simulink model "model3_ReferenceInput"  (R2020a)
settings: Solver=FixedStepAuto  StartTime=0.0  StopTime=T  FixedStep=Ts  RelTol=1e-3
undefined symbols (not defined in the file): K, L, M, N, omgn, R, stepT, Ts, x0
settings Model: Creator=XiaoCY  LastModifiedBy=XiaoCY
settings DataIOCC: ReturnWorkspaceOutputs=off

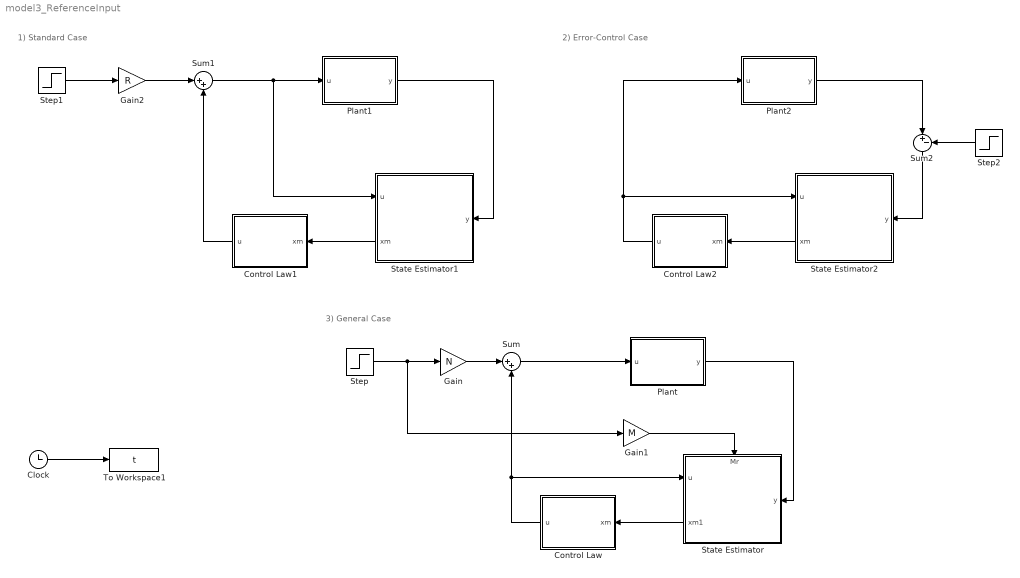
== system model3_ReferenceInput ==
  note: 3) General Case
  note: 1) Standard Case
  note: 2) Error-Control Case
  Clock : Clock
  Control Law : Subsystem
  Control Law1 : Subsystem
  Control Law2 : Subsystem
  Gain : Gain  Gain=N
  Gain1 : Gain  Gain=M
  Gain2 : Gain  Gain=R
  Plant : Subsystem
  Plant1 : Subsystem
  Plant2 : Subsystem
  State Estimator : Subsystem
      settings: PortSchema="{\"entries\":[{\"content\":{\"sides\":[{\"content\":{\"connectorIds\":[\"In1\"]},\"type\":\"ConnectorPlacement.EquallySpacedRectSide\",\"uuid\":\"995efd48-3db5-4a6e-85f6-a349d6a63930\"},{\"content\":{\"connectorIds\":[\"In3\",\"Out1\"],\"side\":\"RIGHT\"},\"type\":\"ConnectorPlacement.EquallySpacedRectSide\",\"uuid\":\"626e22d4-5752-4239-b2ce-472c77ace920\"},{\"content\":{\"connectorIds\":[\"In2\"],\"side\":\"TOP\"},\"type\":\"ConnectorPlacement.EquallySpacedRectSide\",\"uuid\":\"cb599412-420c-4014-940e-49f432b7cbea\"}]},\"type\":\"ConnectorPlacement.EquallySpacedConnector\",\"uuid\":\"e0cccee1-86a0-41f4-a3e5-9044b1b28e69\"}],\"packageUris\":[\"http://schema.mathworks.com/mf0/Connector/19700101\"],\"version\":\"1.0\"}"
  State Estimator1 : Subsystem
      settings: PortSchema="{\"entries\":[{\"content\":{\"sides\":[{\"content\":{\"connectorIds\":[\"In1\"]},\"type\":\"ConnectorPlacement.EquallySpacedRectSide\",\"uuid\":\"995efd48-3db5-4a6e-85f6-a349d6a63930\"},{\"content\":{\"connectorIds\":[\"In2\",\"Out1\"],\"side\":\"RIGHT\"},\"type\":\"ConnectorPlacement.EquallySpacedRectSide\",\"uuid\":\"626e22d4-5752-4239-b2ce-472c77ace920\"},{\"content\":{\"connectorIds\":[],\"side\":\"TOP\"},\"type\":\"ConnectorPlacement.EquallySpacedRectSide\",\"uuid\":\"cb599412-420c-4014-940e-49f432b7cbea\"}]},\"type\":\"ConnectorPlacement.EquallySpacedConnector\",\"uuid\":\"e0cccee1-86a0-41f4-a3e5-9044b1b28e69\"}],\"packageUris\":[\"http://schema.mathworks.com/mf0/Connector/19700101\"],\"version\":\"1.0\"}"
  State Estimator2 : Subsystem
      settings: PortSchema="{\"entries\":[{\"content\":{\"sides\":[{\"content\":{\"connectorIds\":[\"In1\"]},\"type\":\"ConnectorPlacement.EquallySpacedRectSide\",\"uuid\":\"995efd48-3db5-4a6e-85f6-a349d6a63930\"},{\"content\":{\"connectorIds\":[\"In2\",\"Out1\"],\"side\":\"RIGHT\"},\"type\":\"ConnectorPlacement.EquallySpacedRectSide\",\"uuid\":\"626e22d4-5752-4239-b2ce-472c77ace920\"},{\"content\":{\"connectorIds\":[],\"side\":\"TOP\"},\"type\":\"ConnectorPlacement.EquallySpacedRectSide\",\"uuid\":\"cb599412-420c-4014-940e-49f432b7cbea\"}]},\"type\":\"ConnectorPlacement.EquallySpacedConnector\",\"uuid\":\"e0cccee1-86a0-41f4-a3e5-9044b1b28e69\"}],\"packageUris\":[\"http://schema.mathworks.com/mf0/Connector/19700101\"],\"version\":\"1.0\"}"
  Step : Step  Time=stepT  SampleTime=0
  Step1 : Step  Time=stepT  SampleTime=0
  Step2 : Step  Time=stepT  SampleTime=0
  Sum : Sum  Inputs=|++
  Sum1 : Sum  Inputs=|++
  Sum2 : Sum  Inputs=|+-
  To Workspace1 : ToWorkspace  VariableName=t  SampleTime=Ts
  wires:
  Clock/1 -> To Workspace1/1
  Plant/1(y) -> State Estimator/1(y)
  State Estimator/1(xm1) -> Control Law/1(xm)
  Control Law/1(u) -> State Estimator/3(u), Sum/2
  Step/1 -> Gain1/1, Gain/1
  Sum/1 -> Plant/1(u)
  Gain/1 -> Sum/1
  Gain1/1 -> State Estimator/2(Mr)
  Gain2/1 -> Sum1/1
  Sum1/1 -> State Estimator1/2(u), Plant1/1(u)
  Step1/1 -> Gain2/1
  Control Law1/1(u) -> Sum1/2
  State Estimator1/1(xm) -> Control Law1/1(xm)
  Plant1/1(y) -> State Estimator1/1(y)
  State Estimator2/1(xm) -> Control Law2/1(xm)
  Control Law2/1(u) -> Plant2/1(u), State Estimator2/2(u)
  Plant2/1(y) -> Sum2/1
  Sum2/1 -> State Estimator2/1(y)
  Step2/1 -> Sum2/2

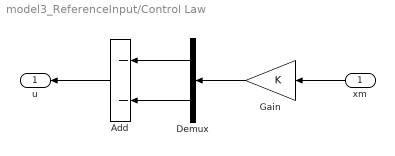
== system model3_ReferenceInput/Control Law ==
  xm : Inport
  Add : Sum  Inputs=--
  Demux : Demux  Outputs=2
  Gain : Gain  Gain=K
  u : Outport
  wires:
  xm/1 -> Gain/1
  Demux/2 -> Add/2
  Add/1 -> u/1
  Gain/1 -> Demux/1
  Demux/1 -> Add/1

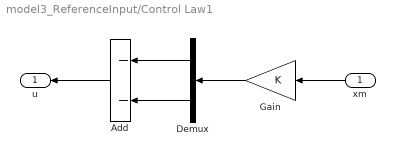
== system model3_ReferenceInput/Control Law1 ==
  xm : Inport
  Add : Sum  Inputs=--
  Demux : Demux  Outputs=2
  Gain : Gain  Gain=K
  u : Outport
  wires:
  Demux/1 -> Add/1
  Gain/1 -> Demux/1
  Add/1 -> u/1
  Demux/2 -> Add/2
  xm/1 -> Gain/1

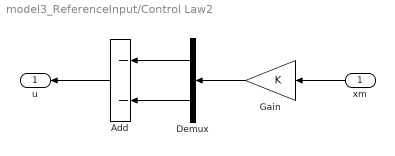
== system model3_ReferenceInput/Control Law2 ==
  xm : Inport
  Add : Sum  Inputs=--
  Demux : Demux  Outputs=2
  Gain : Gain  Gain=K
  u : Outport
  wires:
  xm/1 -> Gain/1
  Demux/2 -> Add/2
  Add/1 -> u/1
  Gain/1 -> Demux/1
  Demux/1 -> Add/1

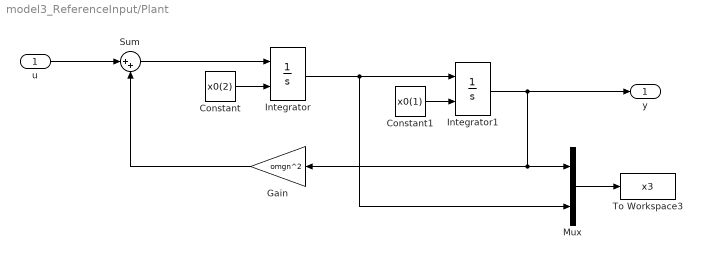
== system model3_ReferenceInput/Plant ==
  u : Inport
  Constant : Constant  Value=x0(2)
  Constant1 : Constant  Value=x0(1)
  Gain : Gain  Gain=omgn^2
  Integrator : Integrator  InitialConditionSource=external
  Integrator1 : Integrator  InitialConditionSource=external
  Mux : Mux  Inputs=2
  Sum : Sum  Inputs=|++
  To Workspace3 : ToWorkspace  VariableName=x3  SampleTime=Ts
  y : Outport
  wires:
  Integrator/1 -> Mux/2, Integrator1/1
  Constant1/1 -> Integrator1/2
  u/1 -> Sum/1
  Constant/1 -> Integrator/2
  Sum/1 -> Integrator/1
  Gain/1 -> Sum/2
  Mux/1 -> To Workspace3/1
  Integrator1/1 -> Gain/1, Mux/1, y/1

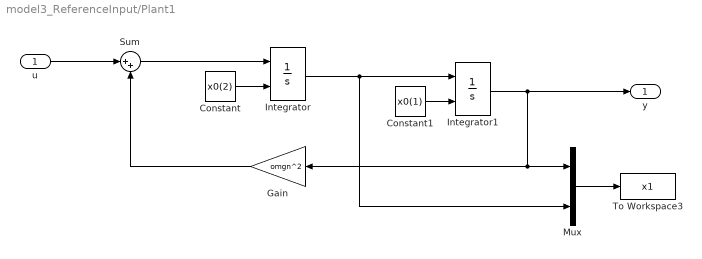
== system model3_ReferenceInput/Plant1 ==
  u : Inport
  Constant : Constant  Value=x0(2)
  Constant1 : Constant  Value=x0(1)
  Gain : Gain  Gain=omgn^2
  Integrator : Integrator  InitialConditionSource=external
  Integrator1 : Integrator  InitialConditionSource=external
  Mux : Mux  Inputs=2
  Sum : Sum  Inputs=|++
  To Workspace3 : ToWorkspace  VariableName=x1  SampleTime=Ts
  y : Outport
  wires:
  Integrator1/1 -> y/1, Mux/1, Gain/1
  Mux/1 -> To Workspace3/1
  Gain/1 -> Sum/2
  Sum/1 -> Integrator/1
  Constant/1 -> Integrator/2
  u/1 -> Sum/1
  Constant1/1 -> Integrator1/2
  Integrator/1 -> Integrator1/1, Mux/2

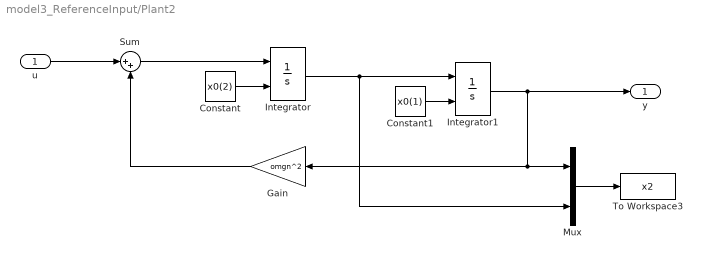
== system model3_ReferenceInput/Plant2 ==
  u : Inport
  Constant : Constant  Value=x0(2)
  Constant1 : Constant  Value=x0(1)
  Gain : Gain  Gain=omgn^2
  Integrator : Integrator  InitialConditionSource=external
  Integrator1 : Integrator  InitialConditionSource=external
  Mux : Mux  Inputs=2
  Sum : Sum  Inputs=|++
  To Workspace3 : ToWorkspace  VariableName=x2  SampleTime=Ts
  y : Outport
  wires:
  Integrator/1 -> Mux/2, Integrator1/1
  Constant1/1 -> Integrator1/2
  u/1 -> Sum/1
  Constant/1 -> Integrator/2
  Sum/1 -> Integrator/1
  Gain/1 -> Sum/2
  Mux/1 -> To Workspace3/1
  Integrator1/1 -> Gain/1, Mux/1, y/1

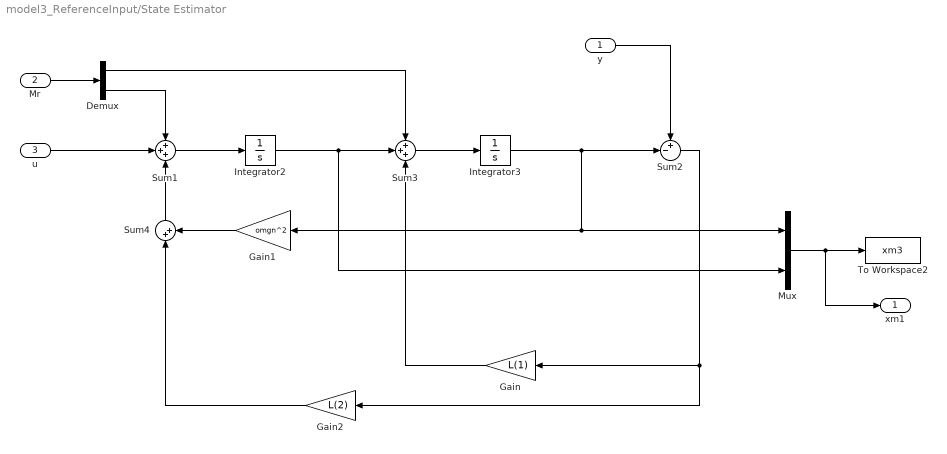
== system model3_ReferenceInput/State Estimator ==
  y : Inport
  Mr : Inport  Port=2
  u : Inport  Port=3
  Demux : Demux  Outputs=2
  Gain : Gain  Gain=L(1)
  Gain1 : Gain  Gain=omgn^2
  Gain2 : Gain  Gain=L(2)
  Integrator2 : Integrator
  Integrator3 : Integrator
  Mux : Mux  Inputs=2
  Sum1 : Sum  Inputs=+++
  Sum2 : Sum  Inputs=+-|
  Sum3 : Sum  Inputs=+++
  Sum4 : Sum  Inputs=|++
  To Workspace2 : ToWorkspace  VariableName=xm3  SampleTime=Ts
  xm1 : Outport
  wires:
  y/1 -> Sum2/1
  Integrator3/1 -> Sum2/2, Mux/1, Gain1/1
  Sum1/1 -> Integrator2/1
  u/1 -> Sum1/2
  Integrator2/1 -> Sum3/2, Mux/2
  Mux/1 -> xm1/1, To Workspace2/1
  Sum2/1 -> Gain2/1, Gain/1
  Sum3/1 -> Integrator3/1
  Gain1/1 -> Sum4/2
  Sum4/1 -> Sum1/3
  Gain/1 -> Sum3/3
  Gain2/1 -> Sum4/1
  Mr/1 -> Demux/1
  Demux/1 -> Sum3/1
  Demux/2 -> Sum1/1

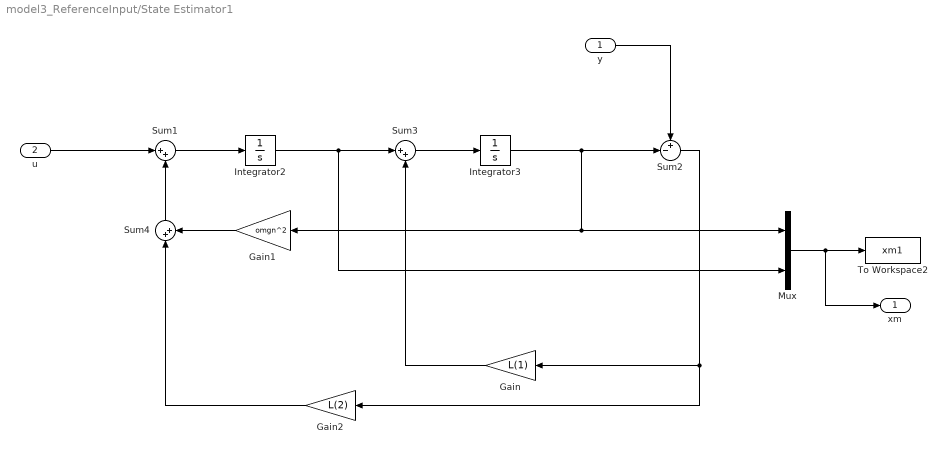
== system model3_ReferenceInput/State Estimator1 ==
  y : Inport
  u : Inport  Port=2
  Gain : Gain  Gain=L(1)
  Gain1 : Gain  Gain=omgn^2
  Gain2 : Gain  Gain=L(2)
  Integrator2 : Integrator
  Integrator3 : Integrator
  Mux : Mux  Inputs=2
  Sum1 : Sum  Inputs=|++
  Sum2 : Sum  Inputs=+-|
  Sum3 : Sum  Inputs=|++
  Sum4 : Sum  Inputs=|++
  To Workspace2 : ToWorkspace  VariableName=xm1  SampleTime=Ts
  xm : Outport
  wires:
  Gain2/1 -> Sum4/1
  Gain/1 -> Sum3/2
  Sum4/1 -> Sum1/2
  Gain1/1 -> Sum4/2
  Sum3/1 -> Integrator3/1
  Sum2/1 -> Gain/1, Gain2/1
  Mux/1 -> To Workspace2/1, xm/1
  Integrator2/1 -> Sum3/1, Mux/2
  u/1 -> Sum1/1
  Sum1/1 -> Integrator2/1
  Integrator3/1 -> Gain1/1, Mux/1, Sum2/2
  y/1 -> Sum2/1

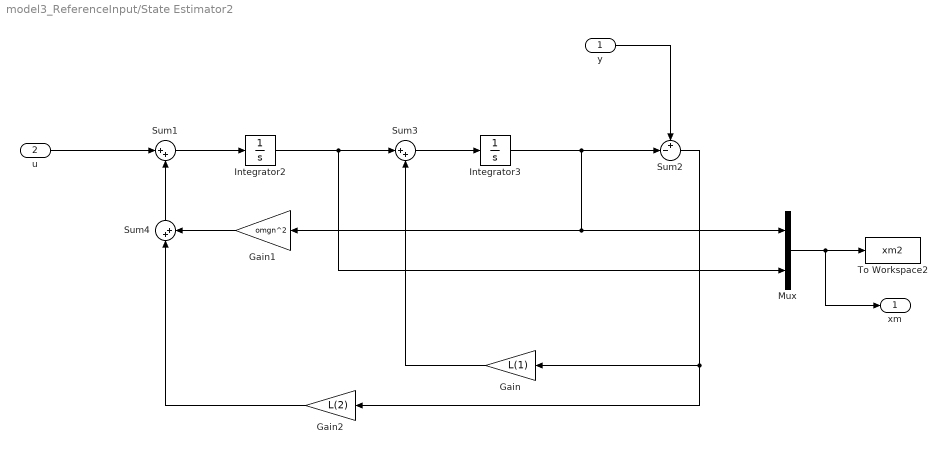
== system model3_ReferenceInput/State Estimator2 ==
  y : Inport
  u : Inport  Port=2
  Gain : Gain  Gain=L(1)
  Gain1 : Gain  Gain=omgn^2
  Gain2 : Gain  Gain=L(2)
  Integrator2 : Integrator
  Integrator3 : Integrator
  Mux : Mux  Inputs=2
  Sum1 : Sum  Inputs=|++
  Sum2 : Sum  Inputs=+-|
  Sum3 : Sum  Inputs=|++
  Sum4 : Sum  Inputs=|++
  To Workspace2 : ToWorkspace  VariableName=xm2  SampleTime=Ts
  xm : Outport
  wires:
  y/1 -> Sum2/1
  Integrator3/1 -> Sum2/2, Mux/1, Gain1/1
  Sum1/1 -> Integrator2/1
  u/1 -> Sum1/1
  Integrator2/1 -> Mux/2, Sum3/1
  Mux/1 -> xm/1, To Workspace2/1
  Sum2/1 -> Gain2/1, Gain/1
  Sum3/1 -> Integrator3/1
  Gain1/1 -> Sum4/2
  Sum4/1 -> Sum1/2
  Gain/1 -> Sum3/2
  Gain2/1 -> Sum4/1
